simulink model "lab_02_fuzzy_alap_simulink_2"  (R2024a)
settings: Solver=VariableStepAuto  StartTime=0.0  StopTime=50  RelTol=1e-3
libraries: fuzblock x1
settings Model: Creator=Admin  LastModifiedBy=Admin

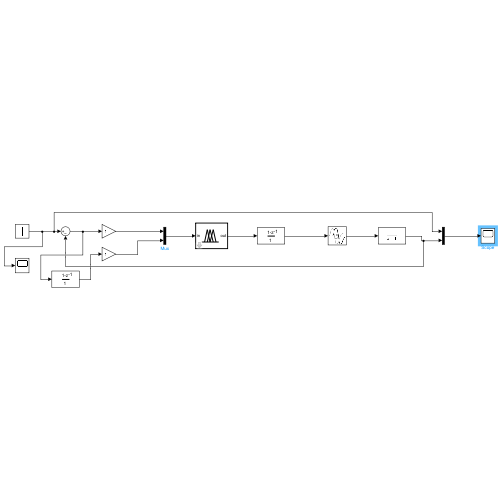
[thumbnail: Simulink's stored preview of the top-level diagram]
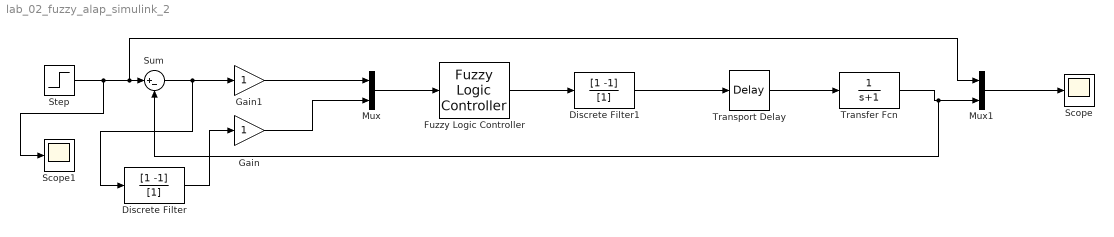
== system lab_02_fuzzy_alap_simulink_2 ==
  Discrete Filter : DiscreteFilter  Numerator=[1 -1]  Denominator=[1]
  Discrete Filter1 : DiscreteFilter  Numerator=[1 -1]  Denominator=[1]
  Fuzzy Logic Controller : fuzblock/Fuzzy Logic  Controller  FIS=mamdanitype1_v2  OutputSampleNumber=101  DataType=double  FuzzifiedInputs=off  RuleFiringStrengths=off  RuleOutputs=off  AggregatedOutputs=off  SimulateUsing=Interpreted execution  OutOfRangeInputValueMessage=warning  NoRuleFiredMessage=warning  EmptyOutputFuzzySetMessage=warning
  Gain : Gain
  Gain1 : Gain
  Mux : Mux  Inputs=2
  Mux1 : Mux  Inputs=2
  Scope : Scope
  Scope1 : Scope
  Step : Step  SampleTime=0
  Sum : Sum  Inputs=|+-
  Transfer Fcn : TransferFcn  Denominator=[1 1]
  Transport Delay : TransportDelay
  wires:
  Mux/1 -> Fuzzy Logic Controller/1
  Step/1 -> Scope1/1, Mux1/1, Sum/1
  Sum/1 -> Discrete Filter/1, Gain1/1
  Discrete Filter/1 -> Gain/1
  Gain/1 -> Mux/2
  Gain1/1 -> Mux/1
  Fuzzy Logic Controller/1 -> Discrete Filter1/1
  Discrete Filter1/1 -> Transport Delay/1
  Transport Delay/1 -> Transfer Fcn/1
  Transfer Fcn/1 -> Sum/2, Mux1/2
  Mux1/1 -> Scope/1
